simulink model "Enable_Triggered_Subsystem"  (R2025b)
settings: Solver=FixedStepDiscrete  StartTime=0.0  StopTime=10.0  FixedStep=0.01  RelTol=1e-3
libraries: simulink x1
settings Model: Creator=soura  LastModifiedBy=soura

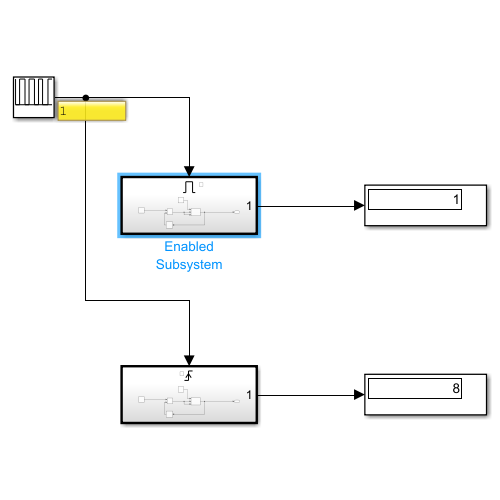
[thumbnail: Simulink's stored preview of the top-level diagram]
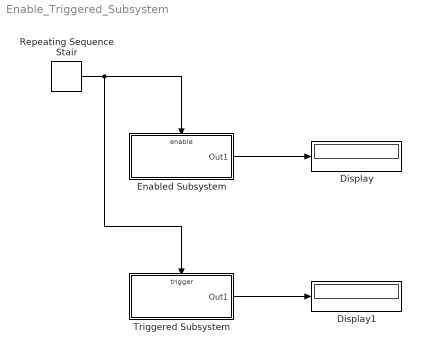
== system Enable_Triggered_Subsystem ==
  Display : Display
  Display1 : Display
  Enabled Subsystem : Subsystem  TreatAsAtomicUnit=on
  Repeating Sequence Stair : simulink/Sources/Repeating Sequence Stair  OutValues=[0 1 0 1 0 1 0 1].'  tsamp=-1  OutMin=[]  OutMax=[]  OutDataTypeStr=double  OutputDataTypeScalingMode=double  OutDataType=fixdt(0,8)  ConRadixGroup=Best Precision: Vector-wise  OutScaling=2^-12
  Triggered Subsystem : Subsystem  TreatAsAtomicUnit=on
  wires:
  Repeating Sequence Stair/1 -> Triggered Subsystem/Trigger, Enabled Subsystem/Enable
  Enabled Subsystem/1(Out1) -> Display/1
  Triggered Subsystem/1(Out1) -> Display1/1

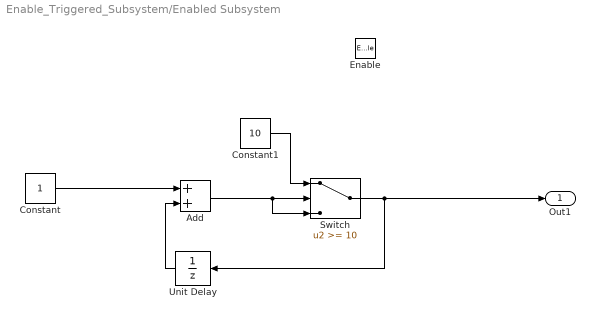
== system Enable_Triggered_Subsystem/Enabled Subsystem ==
  Enable : EnablePort
  Add : Sum
  Constant : Constant
  Constant1 : Constant  Value=10
  Switch : Switch  Threshold=10  SaturateOnIntegerOverflow=off  InputSameDT=off
  Unit Delay : UnitDelay  SampleTime=-1  HasFrameUpgradeWarning=on
  Out1 : Outport  InitialOutput=0
  wires:
  Unit Delay/1 -> Add/2
  Add/1 -> Switch/3, Switch/2
  Constant1/1 -> Switch/1
  Switch/1 -> Out1/1, Unit Delay/1
  Constant/1 -> Add/1

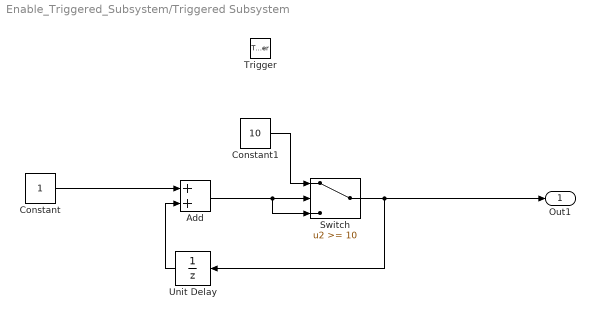
== system Enable_Triggered_Subsystem/Triggered Subsystem ==
  Trigger : TriggerPort  VariantControl=(inherit)
  Add : Sum
  Constant : Constant
  Constant1 : Constant  Value=10
  Switch : Switch  Threshold=10  SaturateOnIntegerOverflow=off  InputSameDT=off
  Unit Delay : UnitDelay  SampleTime=-1  HasFrameUpgradeWarning=on
  Out1 : Outport  InitialOutput=0
  wires:
  Unit Delay/1 -> Add/2
  Switch/1 -> Out1/1, Unit Delay/1
  Constant1/1 -> Switch/1
  Add/1 -> Switch/3, Switch/2
  Constant/1 -> Add/1
